simulink model "Levitatore_lin"  (R2017a)
settings: Solver=ode45  StartTime=0.0  StopTime=t_stop  MaxStep=max_step  MinStep=min_step  RelTol=1e-3
values from neighbouring files (symbols this model uses):
  max_step = 1e-4    (= 0.0001)    [Controllore_loopshaping.m]    (also in Simulazione_lineare.m)
  r_s = -1    [Controllore_loopshaping.m]    (also in Simulazione_lineare.m)
  rho = 0    [Controllore_loopshaping.m]    (also in Simulazione_lineare.m)
  rho_ramp = 1    [Controllore_loopshaping.m]    (also in Simulazione_lineare.m)
  Ts = 1e-3    (= 0.001)    [Controllore_giusto.m]    (also in Controllore_loopshaping.m)
libraries: cstblocks x2, simulink x1
settings Model: Creator=FEDERICA  LastModifiedBy=S234152
settings SolverCC: InitialStep=min_step

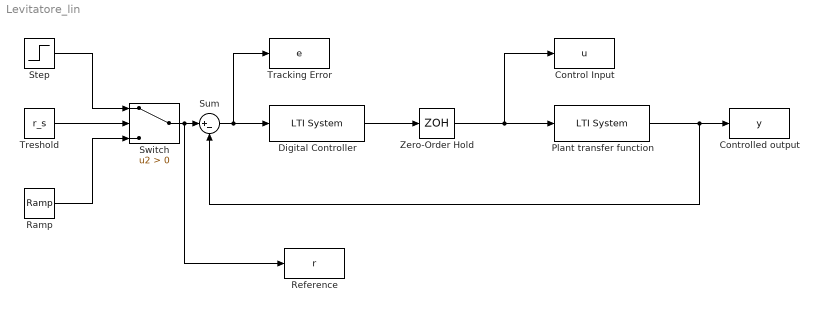
== system Levitatore_lin ==
  Control Input : ToWorkspace  VariableName=u  SaveFormat=Timeseries  SampleTime=max_step
  Controlled output : ToWorkspace  VariableName=y  SaveFormat=Timeseries  SampleTime=max_step
  Digital Controller : cstblocks/LTI System  sys=Cd  IC=[]
  Plant transfer function : cstblocks/LTI System  sys=G1  IC=[]
  Ramp : simulink/Sources/Ramp  slope=rho_ramp  start=0  X0=0
  Reference : ToWorkspace  VariableName=r  SaveFormat=Timeseries  SampleTime=max_step
  Step : Step  Time=0  After=rho  SampleTime=0
  Sum : Sum  Inputs=|+-
  Switch : Switch  Criteria=u2 > Threshold
  Tracking Error : ToWorkspace  VariableName=e  SaveFormat=Timeseries  SampleTime=Ts
  Treshold : Constant  Value=r_s
  Zero-Order Hold : ZeroOrderHold  SampleTime=-1
  wires:
  Zero-Order Hold/1 -> Control Input/1, Plant transfer function/1
  Digital Controller/1 -> Zero-Order Hold/1
  Sum/1 -> Tracking Error/1, Digital Controller/1
  Switch/1 -> Reference/1, Sum/1
  Plant transfer function/1 -> Sum/2, Controlled output/1
  Treshold/1 -> Switch/2
  Step/1 -> Switch/1
  Ramp/1 -> Switch/3
